simulink model "test3_3_model"  (R2018b)
settings: Solver=FixedStepAuto  StartTime=0.0  StopTime=Endtime  FixedStep=smp  RelTol=1e-3
values from neighbouring files (symbols this model uses):
  D = 10    [test3_3.m]
  f = 10    [test3_3.m]
  g = 9.8    [test3_3.m]
  k = 100    [test3_3.m]
  M = 10    [test3_3.m]
  p_cycle = 20    [test3_3.m]
  p_width = 50    [test3_3.m]
  smp = 0.001    [test3_3.m]
settings Model: Creator=nharada  LastModifiedBy=nharada

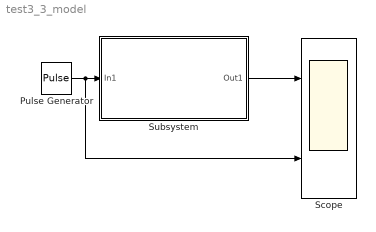
== system test3_3_model ==
  Pulse Generator : DiscretePulseGenerator  PulseType=Time based  Amplitude=f  Period=p_cycle  PulseWidth=p_width  PhaseDelay=10  SampleTime=smp
  Scope : Scope  NumInputPorts=2
  Subsystem : Subsystem
  wires:
  Pulse Generator/1 -> Scope/2, Subsystem/1(In1)
  Subsystem/1(Out1) -> Scope/1

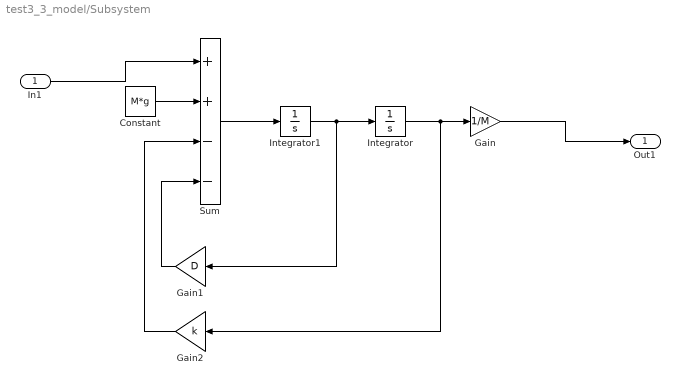
== system test3_3_model/Subsystem ==
  In1 : Inport
  Constant : Constant  Value=M*g
  Gain : Gain  Gain=1/M
  Gain1 : Gain  Gain=D
  Gain2 : Gain  Gain=k
  Integrator : Integrator  InitialCondition=M*g/k
  Integrator1 : Integrator
  Sum : Sum  Inputs=++--
  Out1 : Outport
  wires:
  In1/1 -> Sum/1
  Constant/1 -> Sum/2
  Sum/1 -> Integrator1/1
  Gain/1 -> Out1/1
  Gain2/1 -> Sum/3
  Integrator/1 -> Gain2/1, Gain/1
  Integrator1/1 -> Gain1/1, Integrator/1
  Gain1/1 -> Sum/4
